simulink model "DecoderStepNeuralModel"  (R2016b)
settings: Solver=FixedStepAuto  StartTime=0.0  StopTime=inf  FixedStep=sCoreParams.core.stepPeriod*50  RelTol=1e-3  SampleTimeConstraint=STIndependent  EnableMultiTasking=on
undefined symbols (not defined in the file): neuralModelParams, sCoreParams_neuralModelParams_initialXPre
settings Model: Creator=anish  LastModifiedBy=rzelmann
settings SolverCC: EnableConcurrentExecution=on
settings DataIOCC: SaveFormat=StructureWithTime  SignalLoggingSaveFormat=ModelDataLogs  SaveOutput=off  SignalLogging=off  DSMLogging=off  SaveTime=off
settings OptimizationCC: BlockReduction=off  ConditionallyExecuteInputs=off  DefaultParameterBehavior=Inlined  OptimizeBlockIOStorage=off  BufferReuse=off  GlobalBufferReuse=off  ExpressionFolding=off  LocalBlockOutputs=off  LifeSpan=inf
settings DebuggingCC: SignalRangeChecking=error  SaveWithParameterizedLinksMsg=none  AllowSymbolicDim=off  ModelReferenceSymbolNameMessage=none  StateNameClashWarn=warning  SFUnexpectedBacktrackingDiag=warning  SFNoUnconditionalDefaultTransitionDiag=warning  SFExecutionAtInitializationDiag=none
settings HardwareCC: ProdBitPerPointer=32  ProdBitPerSizeT=32  ProdBitPerPtrDiffT=32  ProdLargestAtomicFloat=None  ProdWordSize=32  ProdLongLongMode=on  ProdHWDeviceType=Generic->32-bit x86 compatible  TargetBitPerPointer=64  TargetLargestAtomicFloat=Float  TargetLongLongMode=on  TargetIntDivRoundTo=Zero  TargetEndianess=LittleEndian  TargetWordSize=64  TargetHWDeviceType=Intel->x86-64 (Windows64)
settings ModelReferenceCC: UpdateModelReferenceTargets=Force  ModelReferenceNumInstancesAllowed=Single  ModelReferencePassRootInputsByReference=off
settings RTWCC: SystemTargetFile=slrt.tlc  TemplateMakefile=slrt_default_tmf  Description=Simulink Real-Time  BuildConfiguration=Faster Runs  RTWCompilerOptimization=on
settings TargetCC: CodeReplacementLibrary=XPC_BLAS  ParMdlRefBuildCompliant=on  ConcurrentExecutionCompliant=on  GeneratePreprocessorConditionals=Use local settings  MatFileLogging=on  MATLABClassNameForMDSCustomization=xpcAperiodicCustomization
settings ConfigComp: CovMetricSettings=dw  CovHtmlReporting=on  CovSaveCumulativeToWorkspaceVar=on  CovSaveSingleToWorkspaceVar=on  CovExternalEMLEnable=off  CovSFcnEnable=off

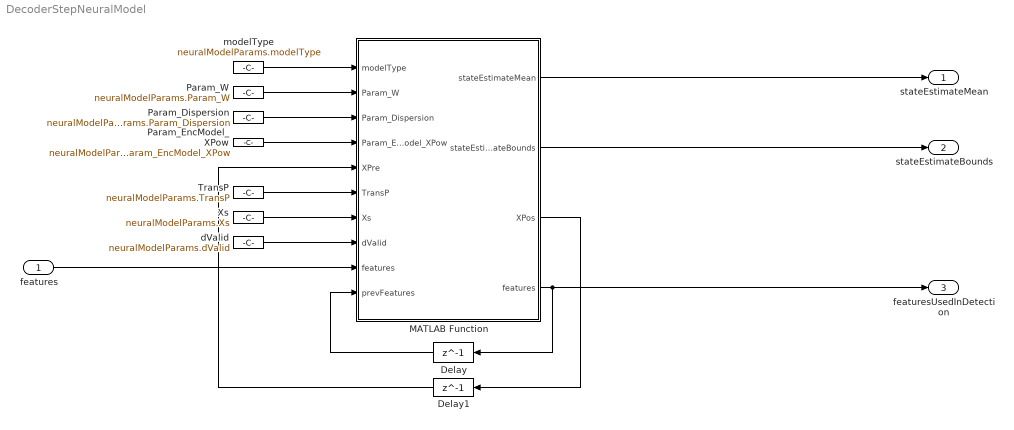
== system DecoderStepNeuralModel ==
  features : Inport  PortDimensions=[1 neuralModelParams.nFeatures]
  Delay : Delay  DelayLength=1
  Delay1 : Delay  DelayLength=1  InitialCondition=sCoreParams_neuralModelParams_initialXPre  InputProcessing=Columns as channels (frame based)
  MATLAB Function : MATLAB Function  TreatAsAtomicUnit=on
  Param_Dispersion : Constant  Value=neuralModelParams.Param_Dispersion
  Param_EncModel_XPow : Constant  Value=neuralModelParams.Param_EncModel_XPow
  Param_W : Constant  Value=neuralModelParams.Param_W
  TransP : Constant  Value=neuralModelParams.TransP
  Xs : Constant  Value=neuralModelParams.Xs
  dValid : Constant  Value=neuralModelParams.dValid
  modelType : Constant  Value=neuralModelParams.modelType
  stateEstimateMean : Outport  InitialOutput=-500
  stateEstimateBounds : Outport  Port=2  InitialOutput=[-500 -500]
  featuresUsedInDetection : Outport  Port=3
  wires:
  MATLAB Function/1(stateEstimateMean) -> stateEstimateMean/1
  MATLAB Function/3(XPos) -> Delay1/1
  dValid/1 -> MATLAB Function/8(dValid)
  Delay/1 -> MATLAB Function/10(prevFeatures)
  modelType/1 -> MATLAB Function/1(modelType)
  Delay1/1 -> MATLAB Function/5(XPre)
  Xs/1 -> MATLAB Function/7(Xs)
  TransP/1 -> MATLAB Function/6(TransP)
  Param_W/1 -> MATLAB Function/2(Param_W)
  Param_Dispersion/1 -> MATLAB Function/3(Param_Dispersion)
  Param_EncModel_XPow/1 -> MATLAB Function/4(Param_EncModel_XPow)
  features/1 -> MATLAB Function/9("features ")
  MATLAB Function/4(features) -> featuresUsedInDetection/1, Delay/1
  MATLAB Function/2(stateEstimateBounds) -> stateEstimateBounds/1

== matlab function DecoderStepNeuralModel/MATLAB Function ==
  data: stateEstimateMean output; stateEstimateBounds output size=[1 2]; modelType input; XPos output; Param_W input; Param_Dispersion input; Param_EncModel_XPow input; XPre input; TransP input; Xs input; dValid input; features output; features input; prevFeatures input
function [stateEstimateMean, stateEstimateBounds, XPos, features] = NeuralModelDecoderDetector(modelType, Param_W, Param_Dispersion, Param_EncModel_XPow, XPre, TransP, Xs, dValid, features, prevFeatures)
%#codegen

% call this per data sample
% modelType: 1= Gamma / 2=Normal (original "model")
% features: is current feature set (original "Yk")
% Yprv: is the feature at previous time (original: "Yprv" - zero at the begining)
% Yk and Yprv have the same length of the features used in the training

% [XPos,CurEstimate] = ay_one_step_decoder(data_type,eParam,XPre,TransP,Xs,dValid,Yk,Yprv);
% XPre = XPos;
% Yprv = Yk;
%avFeatures = zeros(1,length(features)*nEpochs);
%avFeatures = averageFeaturesPerEpoch_EM(features, nEpochs);
%avPrevFeatures = averageFeaturesPerEpoch_EM(prevFeatures, nEpochs);

allFeatures=features(:);

XPos = zeros(1,length(Xs));
stateEstimateMean =0;
TProb = zeros(1,length(Xs));
[XPos, Estimate, TProb]= ay_one_step_decoder_realTime(modelType, Param_W, Param_Dispersion, Param_EncModel_XPow, XPre, TransP, Xs, dValid, allFeatures, prevFeatures);
stateEstimateMean = Estimate.Mean;
stateEstimateBounds = Estimate.Bound;
